simulink model "ROVSim_dp"  (R2020b)
settings: Solver=ode4  StartTime=0.0  StopTime=60  FixedStep=0.05  RelTol=1e-3
InitFcn:
  | initModelParam;
StopFcn:
  | %plotCoupled3DTrack;
libraries: pid_lib x9
settings Model: SimulationMode=accelerator  Creator=53549  LastModifiedBy=53549
settings DataIOCC: ReturnWorkspaceOutputs=off
settings DebuggingCC: ArithmeticOperatorsInVariantConditions=warning
settings SFSimCC: SimUseLocalCustomCode=off  CustomCodeUndefinedFunction=UseInterfaceOnly
settings RTWCC: RTWUseLocalCustomCode=off
settings CodeAppCC: StateflowObjectComments=on

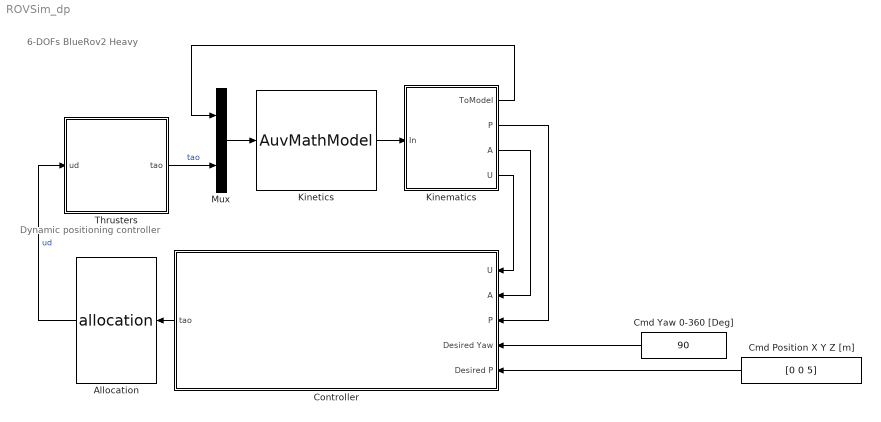
== system ROVSim_dp ==
  note: Dynamic positioning controller
  note: 6-DOFs BlueRov2 Heavy
  Allocation : MATLABFcn  MATLABFcn=allocation  OutputDimensions=8  OutputSignalType=real
  Cmd Position X Y Z [m] : Constant  Value=[0 0 5]
  Cmd Yaw 0-360 [Deg] : Constant  Value=90
  Controller : Subsystem
      mask Display: disp('Controller')
  Kinematics : Subsystem  mask{x0=10.00, y0=-0.00, z0=0.50, pitch0=0, yaw0=154.17, u0=0, flowDir=45, flowVel=0.2}
      mask prompts: x0 "Initiral x"; y0 "Initiral y"; z0 "Initiral z"; pitch0 "Initial pitch [Deg]"; yaw0 "Initial yaw [Deg]"; u0 "Initial velocity [m/s]"; flowDir "Flow direction [Deg]"; flowVel "Flow velocity [m/s]"
      mask DialogControl DescGroupVar Prompt: Kinematics
      mask DialogControl DescTextVar Prompt: Set kinematics information: AMV initial state, flow interference, etc
      mask DialogControl ParameterGroupVar Prompt: Initial state
      mask DialogControl Container3 Prompt: Flow
  Kinetics : MATLABFcn  MATLABFcn=AuvMathModel  OutputDimensions=6  OutputSignalType=real
      mask Display: image('blueRov.jpg')
  Mux : Mux  Inputs=2
  Thrusters : Subsystem  mask{dead_up=0.02, dead_low=-0.02, asym_gain=0.85}
      mask prompts: dead_up "Dead Zone Up Boundary [0, 1]"; dead_low "Dead Zone Low Boundary [-1, 0]"; asym_gain "Asymmetric Gain [0, 1]"
      mask DialogControl DescGroupVar Prompt: Thrusters model
      mask DialogControl DescTextVar Prompt: Thruster dead zone characteristic: When the input is near 0, the thruster does not rotate. Asymmetric characteristics of thrusters: With the same input, the thrust generated by reverse rotation of thrusters is less than that of forward rotation.
      mask Display: image('thruster.jfif');
  wires:
  Kinetics/1 -> Kinematics/1(In)
  Mux/1 -> Kinetics/1
  Kinematics/1(ToModel) -> Mux/1
  Kinematics/2(P) -> Controller/3(P)
  Thrusters/1(tao) -> Mux/2  "tao"
  Cmd Yaw 0-360 [Deg]/1 -> Controller/4(Desired Yaw)
  Cmd Position X Y Z [m]/1 -> Controller/5(Desired P)
  Controller/1(tao) -> Allocation/1
  Allocation/1 -> Thrusters/1(ud)  "ud"
  Kinematics/3(A) -> Controller/2(A)
  Kinematics/4(U) -> Controller/1(U)

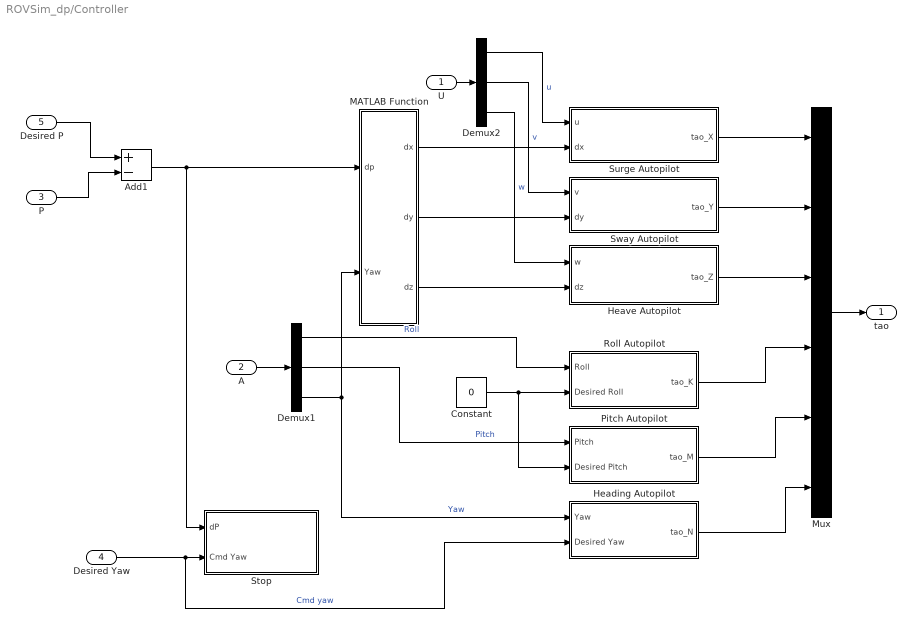
== system ROVSim_dp/Controller ==
  U : Inport
  A : Inport  Port=2
  P : Inport  Port=3
  Desired Yaw : Inport  Port=4
  Desired P : Inport  Port=5
  Add1 : Sum  Inputs=+-
  Constant : Constant  Value=0
  Demux1 : Demux  Outputs=3
  Demux2 : Demux  Outputs=3
  Heading Autopilot : Subsystem  mask{kp=0.2, ki=0, kd=0.2}
      mask DialogControl DescGroupVar Prompt: Heading Autopilot
      mask DialogControl DescTextVar Prompt: 设置PID增益。
      mask DialogControl ParameterGroupVar Prompt: PID Parameter
  Heave Autopilot : Subsystem
  MATLAB Function : MATLAB Function  TreatAsAtomicUnit=on
  Mux : Mux  Inputs=6
  Pitch Autopilot : Subsystem  mask{kp=5, ki=0, kd=0}
      mask DialogControl DescGroupVar Prompt: Heading Autopilot
      mask DialogControl DescTextVar Prompt: 设置PID增益。
      mask DialogControl ParameterGroupVar Prompt: PID Parameter
  Roll Autopilot : Subsystem  mask{kp=5, ki=0, kd=0}
      mask DialogControl DescGroupVar Prompt: Heading Autopilot
      mask DialogControl DescTextVar Prompt: 设置PID增益。
      mask DialogControl ParameterGroupVar Prompt: PID Parameter
  Stop : Subsystem
  Surge Autopilot : Subsystem
  Sway Autopilot : Subsystem
  tao : Outport
  wires:
  Demux1/3 -> Heading Autopilot/1(Yaw), MATLAB Function/2(Yaw)  "Yaw"
  Constant/1 -> Pitch Autopilot/2(Desired Pitch), Roll Autopilot/2(Desired Roll)
  Demux1/2 -> Pitch Autopilot/1(Pitch)  "Pitch"
  A/1 -> Demux1/1
  Desired P/1 -> Add1/1
  Add1/1 -> MATLAB Function/1(dp), Stop/1(dP)
  P/1 -> Add1/2
  Roll Autopilot/1(tao_K) -> Mux/4
  Pitch Autopilot/1(tao_M) -> Mux/5
  Heading Autopilot/1(tao_N) -> Mux/6
  Mux/1 -> tao/1
  Demux1/1 -> Roll Autopilot/1(Roll)  "Roll"
  U/1 -> Demux2/1
  Demux2/1 -> Surge Autopilot/1(u)  "u"
  MATLAB Function/1(dx) -> Surge Autopilot/2(dx)
  Surge Autopilot/1(tao_X) -> Mux/1
  Demux2/2 -> Sway Autopilot/1(v)  "v"
  MATLAB Function/2(dy) -> Sway Autopilot/2(dy)
  Sway Autopilot/1(tao_Y) -> Mux/2
  Demux2/3 -> Heave Autopilot/1(w)  "w"
  MATLAB Function/3(dz) -> Heave Autopilot/2(dz)
  Heave Autopilot/1(tao_Z) -> Mux/3
  Desired Yaw/1 -> Heading Autopilot/2(Desired Yaw), Stop/2(Cmd Yaw)  "Cmd yaw"

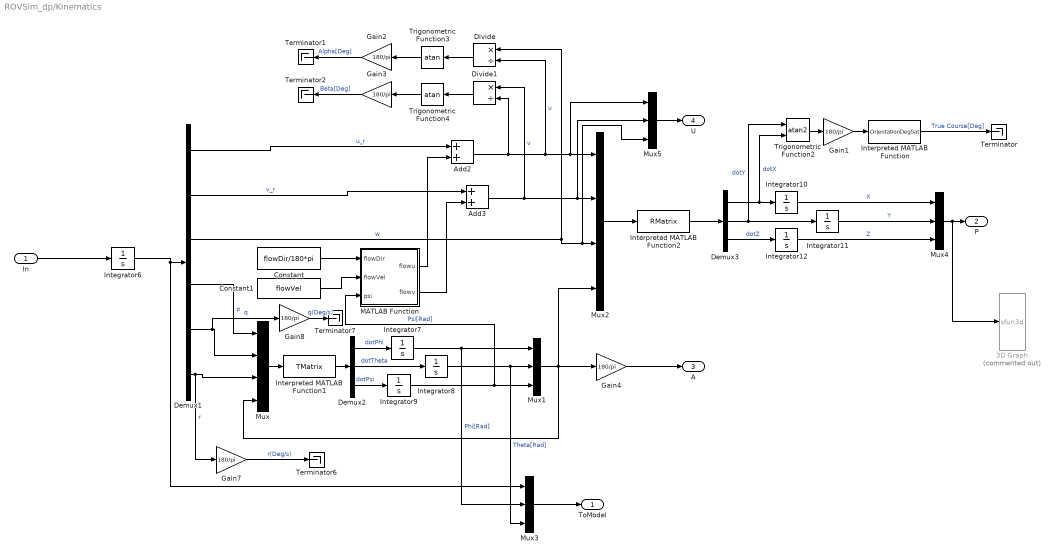
== system ROVSim_dp/Kinematics ==
  In : Inport
  3D Graph : S-Function  Commented=on  LoadFcn=if exist('sfun3d','file'), sfun3d([],[],[],'LoadBlock'); end  FunctionName=sfun3d  Parameters=ax,T,np,cp,gd,ls,mk,mx,hd,tb  SFunctionDeploymentMode=off  EnableBusSupport=off  mask(3D Graph){np=1, ax=[-15 15 -15 15 -5 20], mx=1e4, T=0.1, cp=[3 2 1], gd=on, hd=on, tb=off, ls=-, mk=none}
      mask prompts: np "Number of moving points (lines)"; ax "Range: [xmin xmax  ymin ymax zmin zmax]"; mx "Max number of points in each line"; T "Sampling Time"; cp "Camera position (use [0 0 1] for 2D XY view)"; gd "Grid (on|off)"; hd "HeadMarkers (on|off)"; tb "Toolbar (on|off)"; ls "LineStyle"; mk "LineMarker"
      mask help:
      | This block plots the position of several points in the XYZ space. The input contains the coordinates of all the points (x1,y1,z1,x2,y2,z2,...).
      | The number of moving points (lines), the XYZ ranges, sampling time, camera position, and grid (among other things) can be set as mask parameters.
      settings: CopyFcn=if exist('sfun3d','file'), sfun3d([],[],[],'CopyBlock'); end  DeleteFcn=if exist('sfun3d','file'), sfun3d([],[],[],'DeleteBlock'); end  NameChangeFcn=if exist('sfun3d','file'), sfun3d([],[],[],'NameChange'); end
      mask Help:
      | This block plots the position of several points in the XYZ space. The input contains the coordinates of all the points (x1,y1,z1,x2,y2,z2,...).
      | The number of moving points (lines), the XYZ ranges, sampling time, camera position, and grid (among other things) can be set as mask parameters.
      mask TypeOptions ls: - | -- | : | -. | none
      mask TypeOptions mk: none | . | + | o | * | x | square | diamond | v | ^ | > | < | pentagram | hexagram
      mask Display: plot([.05 .95 .95 .05 .05],[.45 .45 .95 .95 .45], 0.5+cos(0:0.1:2*pi)*0.3,0.7+sin(0:0.1:2*pi)*0.2)
  Add2 : Sum
  Add3 : Sum
  Constant : Constant  Value=flowDir/180*pi
  Constant1 : Constant  Value=flowVel
  Demux1 : Demux  Outputs=6
  Demux2 : Demux  Outputs=3
  Demux3 : Demux  Outputs=3
  Divide : Product  Inputs=*/
  Divide1 : Product  Inputs=*/
  Gain{1..4,7..8} (6 alike) : Gain  Gain=180/pi
  Integrator10 : Integrator  InitialCondition=x0
  Integrator11 : Integrator  InitialCondition=y0
  Integrator12 : Integrator  InitialCondition=z0
  Integrator6 : Integrator  InitialCondition=[u0; 0; 0; 0; 0; 0]
  Integrator7 : Integrator
  Integrator8 : Integrator
  Integrator9 : Integrator  InitialCondition=yaw0*pi/180  WrapState=on  WrappedStateUpperValue=6.2832  WrappedStateLowerValue=0
  Interpreted MATLAB Function : MATLABFcn  MATLABFcn=OrientationDegSat
  Interpreted MATLAB Function1 : MATLABFcn  MATLABFcn=TMatrix  OutputDimensions=3
  Interpreted MATLAB Function2 : MATLABFcn  MATLABFcn=RMatrix  OutputDimensions=3
  MATLAB Function : MATLAB Function  TreatAsAtomicUnit=on
  Mux : Mux
  Mux{1,3..5} (4 alike) : Mux  Inputs=3
  Mux2 : Mux
  Terminator{,1..2,6..7} (5 alike) : Terminator
  Trigonometric Function2 : Trigonometry  Operator=atan2
  Trigonometric Function3 : Trigonometry  Operator=atan
  Trigonometric Function4 : Trigonometry  Operator=atan
  ToModel : Outport
  P : Outport  Port=2
  A : Outport  Port=3
  U : Outport  Port=4
  wires:
  Constant/1 -> MATLAB Function/1(flowDir)
  Constant1/1 -> MATLAB Function/2(flowVel)
  Integrator6/1 -> Mux3/1, Demux1/1
  Demux1/4 -> Mux/1  "p"
  Demux1/5 -> Gain8/1, Mux/2  "q"
  Demux1/6 -> Gain7/1, Mux/3  "r"
  Mux/1 -> Interpreted MATLAB Function1/1
  Interpreted MATLAB Function1/1 -> Demux2/1
  Demux2/1 -> Integrator7/1  "dotPhi"
  Demux2/2 -> Integrator8/1  "dotTheta"
  Demux2/3 -> Integrator9/1  "dotPsi"
  Integrator9/1 -> MATLAB Function/3(psi), Mux1/3  "Psi[Rad]"
  Integrator7/1 -> Mux1/1, Mux3/2  "Phi[Rad]"
  Integrator8/1 -> Mux3/3, Mux1/2  "Theta[Rad]"
  Mux1/1 -> Gain4/1, Mux/4, Mux2/4
  Demux1/1 -> Add2/1  "u_r"
  Demux1/2 -> Add3/1  "v_r"
  Demux1/3 -> Mux5/3, Mux2/3, Divide/1  "w"
  Mux2/1 -> Interpreted MATLAB Function2/1
  Interpreted MATLAB Function2/1 -> Demux3/1
  Demux3/1 -> Trigonometric Function2/2, Integrator10/1  "dotX"
  Demux3/2 -> Trigonometric Function2/1, Integrator11/1  "dotY"
  Demux3/3 -> Integrator12/1  "dotZ"
  Integrator10/1 -> Mux4/1  "X"
  Integrator11/1 -> Mux4/2  "Y"
  Integrator12/1 -> Mux4/3  "Z"
  Gain2/1 -> Terminator1/1  "Alpha[Deg]"
  Trigonometric Function3/1 -> Gain2/1
  Divide/1 -> Trigonometric Function3/1
  Divide1/1 -> Trigonometric Function4/1
  Trigonometric Function4/1 -> Gain3/1
  Gain3/1 -> Terminator2/1  "Beta[Deg]"
  Gain1/1 -> Interpreted MATLAB Function/1
  Interpreted MATLAB Function/1 -> Terminator/1  "True Course[Deg]"
  Trigonometric Function2/1 -> Gain1/1
  Add2/1 -> Divide1/2, Divide/2, Mux5/1, Mux2/1  "u"
  Add3/1 -> Mux5/2, Mux2/2, Divide1/1  "v"
  MATLAB Function/1(flowu) -> Add2/2
  MATLAB Function/2(flowv) -> Add3/2
  Mux3/1 -> ToModel/1
  Mux4/1 -> 3D Graph/1, P/1
  In/1 -> Integrator6/1
  Gain7/1 -> Terminator6/1  "r(Deg/s)"
  Gain8/1 -> Terminator7/1  "q(Deg/s)"
  Gain4/1 -> A/1
  Mux5/1 -> U/1

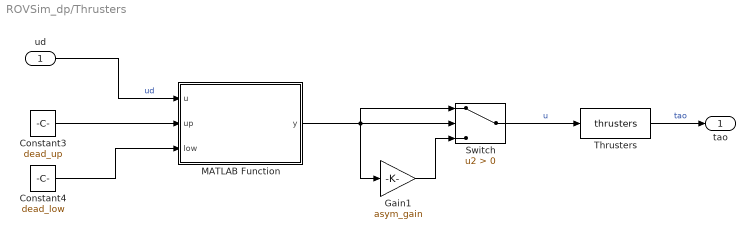
== system ROVSim_dp/Thrusters ==
  ud : Inport
  Constant3 : Constant  Value=dead_up
  Constant4 : Constant  Value=dead_low
  Gain1 : Gain  Gain=asym_gain
  MATLAB Function : MATLAB Function  TreatAsAtomicUnit=on
  Switch : Switch  Criteria=u2 > Threshold
  Thrusters : MATLABFcn  MATLABFcn=thrusters  OutputDimensions=6  OutputSignalType=real
  tao : Outport
  wires:
  Thrusters/1 -> tao/1  "tao"
  ud/1 -> MATLAB Function/1(u)  "ud"
  Gain1/1 -> Switch/3
  MATLAB Function/1(y) -> Switch/1, Gain1/1, Switch/2
  Constant4/1 -> MATLAB Function/3(low)
  Switch/1 -> Thrusters/1  "u"
  Constant3/1 -> MATLAB Function/2(up)

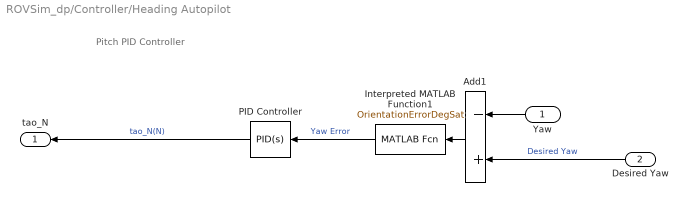
== system ROVSim_dp/Controller/Heading Autopilot ==
  note: Pitch PID Controller
  Yaw : Inport
  Desired Yaw : Inport  Port=2
  Add1 : Sum  Inputs=-+
  Interpreted MATLAB Function1 : MATLABFcn  MATLABFcn=OrientationErrorDegSat  OutputDimensions=1
  PID Controller : pid_lib/PID Controller  Controller=PID  Form=Parallel  TimeDomain=Continuous-time  UseExternalTs=off  SampleTime=-1  IntegratorMethod=Forward Euler  FilterMethod=Forward Euler  ControllerParametersSource=internal  P=kp  I=ki  D=kd  UseFilter=on  N=10  TunerSelectOption=Transfer Function Based (PID Tuner App)  InitialConditionSource=internal  InitialConditionForIntegrator=0  InitialConditionForFilter=0  DifferentiatorICPrevScaledInput=0  ExternalReset=none  TrackingMode=off  Kt=1  LimitOutput=on  SatLimitsSource=internal  UpperSaturationLimit=20  LowerSaturationLimit=-20  LinearizeAsGain=on  AntiWindupMode=none  Kb=1  POutMin=[]  POutMax=[]  IOutMin=[]  IOutMax=[]  DOutMin=[]  DOutMax=[]  NOutMin=[]  NOutMax=[]  SumOutMin=[]  SumOutMax=[]  SaturationOutMin=[]  SaturationOutMax=[]  PParamMin=[]  PParamMax=[]  IParamMin=[]  IParamMax=[]  DParamMin=[]  DParamMax=[]  NParamMin=[]  NParamMax=[]  KbParamMin=[]  KbParamMax=[]  KtParamMin=[]  KtParamMax=[]  KbOutMin=[]  KbOutMax=[]  KtOutMin=[]  KtOutMax=[]  IntegratorOutMin=[]  IntegratorOutMax=[]  FilterOutMin=[]  FilterOutMax=[]  SumI1OutMin=[]  SumI1OutMax=[]  SumI2OutMin=[]  SumI2OutMax=[]  SumI3OutMin=[]  SumI3OutMax=[]  SumI4OutMin=[]  SumI4OutMax=[]  SumDOutMin=[]  SumDOutMax=[]  DifferentiatorOutMin=[]  DifferentiatorOutMax=[]  FilterDiffOutCoefMin=[]  FilterDiffOutCoefMax=[]  ReciprocalOutMin=[]  ReciprocalOutMax=[]  SumDenOutMin=[]  SumDenOutMax=[]  SumNumOutMin=[]  SumNumOutMax=[]  DivideOutMin=[]  DivideOutMax=[]  UdiffTsProdOutMin=[]  UdiffTsProdOutMax=[]  NTsProdOutMin=[]  NTsProdOutMax=[]  UintegralTsProdOutMin=[]  UintegralTsProdOutMax=[]  UngainTsProdOutMin=[]  UngainTsProdOutMax=[]  IntegratorContinuousStateAttributes=''  IntegratorStateMustResolveToSignalObject=off  IntegratorRTWStateStorageClass=Auto  FilterContinuousStateAttributes=''  FilterStateMustResolveToSignalObject=off  FilterRTWStateStorageClass=Auto  ParallelPVariant=InternalParameters  IdealPVariant=Disabled  IVariant=InternalParameters  DVariant=InternalParameters  IntegratorVariant=Continuous  SatVariant=Enabled  AWVariant=Passthrough  PCopyVariant=Disabled  TRVariant=Disabled  FdbkBlocksVariant=Forward  IdealPFdbkVariant=Disabled  SatFdbkVariant=Disabled  DerivativeFilterVariant=ContFilter  NVariant=InternalParameters  NCopyVariant=Disabled  FilterICVariant=InternalICsFilter  IntegratorICVariant=InternalICs  ExternalResetVariant=Disabled  TRSumVariant=Passthrough  SumFdbkVariant=Disabled  SumVariant=Sum_PID  TsampFilterVariant=InternalTs  TsampNgainVariant=Passthrough  TsampIntegralVariant=Passthrough  ExternalSaturationOutDataTypeStr=Inherit: Same as second input
  tao_N : Outport
  wires:
  Yaw/1 -> Add1/1
  PID Controller/1 -> tao_N/1  "tao_N(N)"
  Add1/1 -> Interpreted MATLAB Function1/1
  Desired Yaw/1 -> Add1/2  "Desired Yaw"
  Interpreted MATLAB Function1/1 -> PID Controller/1  "Yaw Error"

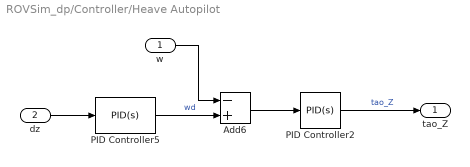
== system ROVSim_dp/Controller/Heave Autopilot ==
  w : Inport
  dz : Inport  Port=2
  Add6 : Sum  Inputs=-+
  PID Controller2 : pid_lib/PID Controller  Controller=PID  Form=Parallel  TimeDomain=Continuous-time  UseExternalTs=off  SampleTime=-1  IntegratorMethod=Forward Euler  FilterMethod=Forward Euler  ControllerParametersSource=internal  P=40  I=0.5  D=0  UseFilter=on  N=100  TunerSelectOption=Transfer Function Based (PID Tuner App)  InitialConditionSource=internal  InitialConditionForIntegrator=0  InitialConditionForFilter=0  DifferentiatorICPrevScaledInput=0  ExternalReset=none  TrackingMode=off  Kt=1  LimitOutput=off  SatLimitsSource=internal  UpperSaturationLimit=inf  LowerSaturationLimit=-inf  LinearizeAsGain=on  AntiWindupMode=none  Kb=1  POutMin=[]  POutMax=[]  IOutMin=[]  IOutMax=[]  DOutMin=[]  DOutMax=[]  NOutMin=[]  NOutMax=[]  SumOutMin=[]  SumOutMax=[]  SaturationOutMin=[]  SaturationOutMax=[]  PParamMin=[]  PParamMax=[]  IParamMin=[]  IParamMax=[]  DParamMin=[]  DParamMax=[]  NParamMin=[]  NParamMax=[]  KbParamMin=[]  KbParamMax=[]  KtParamMin=[]  KtParamMax=[]  KbOutMin=[]  KbOutMax=[]  KtOutMin=[]  KtOutMax=[]  IntegratorOutMin=[]  IntegratorOutMax=[]  FilterOutMin=[]  FilterOutMax=[]  SumI1OutMin=[]  SumI1OutMax=[]  SumI2OutMin=[]  SumI2OutMax=[]  SumI3OutMin=[]  SumI3OutMax=[]  SumI4OutMin=[]  SumI4OutMax=[]  SumDOutMin=[]  SumDOutMax=[]  DifferentiatorOutMin=[]  DifferentiatorOutMax=[]  FilterDiffOutCoefMin=[]  FilterDiffOutCoefMax=[]  ReciprocalOutMin=[]  ReciprocalOutMax=[]  SumDenOutMin=[]  SumDenOutMax=[]  SumNumOutMin=[]  SumNumOutMax=[]  DivideOutMin=[]  DivideOutMax=[]  UdiffTsProdOutMin=[]  UdiffTsProdOutMax=[]  NTsProdOutMin=[]  NTsProdOutMax=[]  UintegralTsProdOutMin=[]  UintegralTsProdOutMax=[]  UngainTsProdOutMin=[]  UngainTsProdOutMax=[]  IntegratorContinuousStateAttributes=''  IntegratorStateMustResolveToSignalObject=off  IntegratorRTWStateStorageClass=Auto  FilterContinuousStateAttributes=''  FilterStateMustResolveToSignalObject=off  FilterRTWStateStorageClass=Auto  ParallelPVariant=InternalParameters  IdealPVariant=Disabled  IVariant=InternalParameters  DVariant=InternalParameters  IntegratorVariant=Continuous  SatVariant=Disabled  AWVariant=Passthrough  PCopyVariant=Disabled  TRVariant=Disabled  FdbkBlocksVariant=Forward  IdealPFdbkVariant=Disabled  SatFdbkVariant=Disabled  DerivativeFilterVariant=ContFilter  NVariant=InternalParameters  NCopyVariant=Disabled  FilterICVariant=InternalICsFilter  IntegratorICVariant=InternalICs  ExternalResetVariant=Disabled  TRSumVariant=Passthrough  SumFdbkVariant=Disabled  SumVariant=Sum_PID  TsampFilterVariant=InternalTs  TsampNgainVariant=Passthrough  TsampIntegralVariant=Passthrough  ExternalSaturationOutDataTypeStr=Inherit: Same as second input
  PID Controller5 : pid_lib/PID Controller  Controller=PID  Form=Parallel  TimeDomain=Continuous-time  UseExternalTs=off  SampleTime=-1  IntegratorMethod=Forward Euler  FilterMethod=Forward Euler  ControllerParametersSource=internal  P=0.5  I=0  D=0  UseFilter=on  N=100  TunerSelectOption=Transfer Function Based (PID Tuner App)  InitialConditionSource=internal  InitialConditionForIntegrator=0  InitialConditionForFilter=0  DifferentiatorICPrevScaledInput=0  ExternalReset=none  TrackingMode=off  Kt=1  LimitOutput=on  SatLimitsSource=internal  UpperSaturationLimit=1  LowerSaturationLimit=-1  LinearizeAsGain=on  AntiWindupMode=none  Kb=1  POutMin=[]  POutMax=[]  IOutMin=[]  IOutMax=[]  DOutMin=[]  DOutMax=[]  NOutMin=[]  NOutMax=[]  SumOutMin=[]  SumOutMax=[]  SaturationOutMin=[]  SaturationOutMax=[]  PParamMin=[]  PParamMax=[]  IParamMin=[]  IParamMax=[]  DParamMin=[]  DParamMax=[]  NParamMin=[]  NParamMax=[]  KbParamMin=[]  KbParamMax=[]  KtParamMin=[]  KtParamMax=[]  KbOutMin=[]  KbOutMax=[]  KtOutMin=[]  KtOutMax=[]  IntegratorOutMin=[]  IntegratorOutMax=[]  FilterOutMin=[]  FilterOutMax=[]  SumI1OutMin=[]  SumI1OutMax=[]  SumI2OutMin=[]  SumI2OutMax=[]  SumI3OutMin=[]  SumI3OutMax=[]  SumI4OutMin=[]  SumI4OutMax=[]  SumDOutMin=[]  SumDOutMax=[]  DifferentiatorOutMin=[]  DifferentiatorOutMax=[]  FilterDiffOutCoefMin=[]  FilterDiffOutCoefMax=[]  ReciprocalOutMin=[]  ReciprocalOutMax=[]  SumDenOutMin=[]  SumDenOutMax=[]  SumNumOutMin=[]  SumNumOutMax=[]  DivideOutMin=[]  DivideOutMax=[]  UdiffTsProdOutMin=[]  UdiffTsProdOutMax=[]  NTsProdOutMin=[]  NTsProdOutMax=[]  UintegralTsProdOutMin=[]  UintegralTsProdOutMax=[]  UngainTsProdOutMin=[]  UngainTsProdOutMax=[]  IntegratorContinuousStateAttributes=''  IntegratorStateMustResolveToSignalObject=off  IntegratorRTWStateStorageClass=Auto  FilterContinuousStateAttributes=''  FilterStateMustResolveToSignalObject=off  FilterRTWStateStorageClass=Auto  ParallelPVariant=InternalParameters  IdealPVariant=Disabled  IVariant=InternalParameters  DVariant=InternalParameters  IntegratorVariant=Continuous  SatVariant=Enabled  AWVariant=Passthrough  PCopyVariant=Disabled  TRVariant=Disabled  FdbkBlocksVariant=Forward  IdealPFdbkVariant=Disabled  SatFdbkVariant=Disabled  DerivativeFilterVariant=ContFilter  NVariant=InternalParameters  NCopyVariant=Disabled  FilterICVariant=InternalICsFilter  IntegratorICVariant=InternalICs  ExternalResetVariant=Disabled  TRSumVariant=Passthrough  SumFdbkVariant=Disabled  SumVariant=Sum_PID  TsampFilterVariant=InternalTs  TsampNgainVariant=Passthrough  TsampIntegralVariant=Passthrough  ExternalSaturationOutDataTypeStr=Inherit: Same as second input
  tao_Z : Outport
  wires:
  Add6/1 -> PID Controller2/1
  PID Controller5/1 -> Add6/2  "wd"
  dz/1 -> PID Controller5/1
  PID Controller2/1 -> tao_Z/1  "tao_Z"
  w/1 -> Add6/1

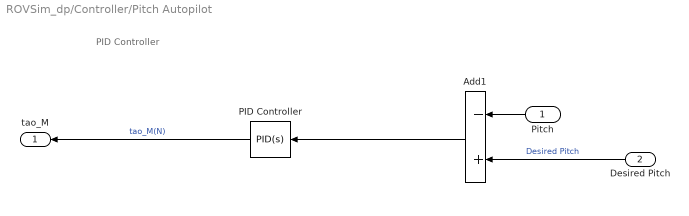
== system ROVSim_dp/Controller/Pitch Autopilot ==
  note: PID Controller
  Pitch : Inport
  Desired Pitch : Inport  Port=2
  Add1 : Sum  Inputs=-+
  PID Controller : pid_lib/PID Controller  Controller=PID  Form=Parallel  TimeDomain=Continuous-time  UseExternalTs=off  SampleTime=-1  IntegratorMethod=Forward Euler  FilterMethod=Forward Euler  ControllerParametersSource=internal  P=kp  I=ki  D=kd  UseFilter=on  N=10  TunerSelectOption=Transfer Function Based (PID Tuner App)  InitialConditionSource=internal  InitialConditionForIntegrator=0  InitialConditionForFilter=0  DifferentiatorICPrevScaledInput=0  ExternalReset=none  TrackingMode=off  Kt=1  LimitOutput=on  SatLimitsSource=internal  UpperSaturationLimit=20  LowerSaturationLimit=-20  LinearizeAsGain=on  AntiWindupMode=none  Kb=1  POutMin=[]  POutMax=[]  IOutMin=[]  IOutMax=[]  DOutMin=[]  DOutMax=[]  NOutMin=[]  NOutMax=[]  SumOutMin=[]  SumOutMax=[]  SaturationOutMin=[]  SaturationOutMax=[]  PParamMin=[]  PParamMax=[]  IParamMin=[]  IParamMax=[]  DParamMin=[]  DParamMax=[]  NParamMin=[]  NParamMax=[]  KbParamMin=[]  KbParamMax=[]  KtParamMin=[]  KtParamMax=[]  KbOutMin=[]  KbOutMax=[]  KtOutMin=[]  KtOutMax=[]  IntegratorOutMin=[]  IntegratorOutMax=[]  FilterOutMin=[]  FilterOutMax=[]  SumI1OutMin=[]  SumI1OutMax=[]  SumI2OutMin=[]  SumI2OutMax=[]  SumI3OutMin=[]  SumI3OutMax=[]  SumI4OutMin=[]  SumI4OutMax=[]  SumDOutMin=[]  SumDOutMax=[]  DifferentiatorOutMin=[]  DifferentiatorOutMax=[]  FilterDiffOutCoefMin=[]  FilterDiffOutCoefMax=[]  ReciprocalOutMin=[]  ReciprocalOutMax=[]  SumDenOutMin=[]  SumDenOutMax=[]  SumNumOutMin=[]  SumNumOutMax=[]  DivideOutMin=[]  DivideOutMax=[]  UdiffTsProdOutMin=[]  UdiffTsProdOutMax=[]  NTsProdOutMin=[]  NTsProdOutMax=[]  UintegralTsProdOutMin=[]  UintegralTsProdOutMax=[]  UngainTsProdOutMin=[]  UngainTsProdOutMax=[]  IntegratorContinuousStateAttributes=''  IntegratorStateMustResolveToSignalObject=off  IntegratorRTWStateStorageClass=Auto  FilterContinuousStateAttributes=''  FilterStateMustResolveToSignalObject=off  FilterRTWStateStorageClass=Auto  ParallelPVariant=InternalParameters  IdealPVariant=Disabled  IVariant=InternalParameters  DVariant=InternalParameters  IntegratorVariant=Continuous  SatVariant=Enabled  AWVariant=Passthrough  PCopyVariant=Disabled  TRVariant=Disabled  FdbkBlocksVariant=Forward  IdealPFdbkVariant=Disabled  SatFdbkVariant=Disabled  DerivativeFilterVariant=ContFilter  NVariant=InternalParameters  NCopyVariant=Disabled  FilterICVariant=InternalICsFilter  IntegratorICVariant=InternalICs  ExternalResetVariant=Disabled  TRSumVariant=Passthrough  SumFdbkVariant=Disabled  SumVariant=Sum_PID  TsampFilterVariant=InternalTs  TsampNgainVariant=Passthrough  TsampIntegralVariant=Passthrough  ExternalSaturationOutDataTypeStr=Inherit: Same as second input
  tao_M : Outport
  wires:
  Add1/1 -> PID Controller/1
  Desired Pitch/1 -> Add1/2  "Desired Pitch"
  PID Controller/1 -> tao_M/1  "tao_M(N)"
  Pitch/1 -> Add1/1

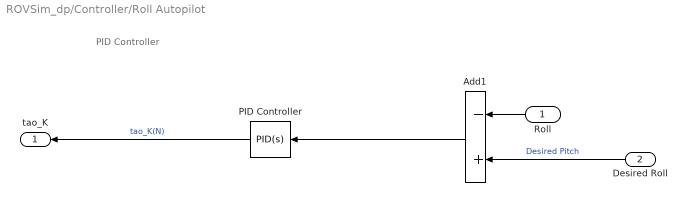
== system ROVSim_dp/Controller/Roll Autopilot ==
  note: PID Controller
  Roll : Inport
  Desired Roll : Inport  Port=2
  Add1 : Sum  Inputs=-+
  PID Controller : pid_lib/PID Controller  Controller=PID  Form=Parallel  TimeDomain=Continuous-time  UseExternalTs=off  SampleTime=-1  IntegratorMethod=Forward Euler  FilterMethod=Forward Euler  ControllerParametersSource=internal  P=kp  I=ki  D=kd  UseFilter=on  N=10  TunerSelectOption=Transfer Function Based (PID Tuner App)  InitialConditionSource=internal  InitialConditionForIntegrator=0  InitialConditionForFilter=0  DifferentiatorICPrevScaledInput=0  ExternalReset=none  TrackingMode=off  Kt=1  LimitOutput=on  SatLimitsSource=internal  UpperSaturationLimit=20  LowerSaturationLimit=-20  LinearizeAsGain=on  AntiWindupMode=none  Kb=1  POutMin=[]  POutMax=[]  IOutMin=[]  IOutMax=[]  DOutMin=[]  DOutMax=[]  NOutMin=[]  NOutMax=[]  SumOutMin=[]  SumOutMax=[]  SaturationOutMin=[]  SaturationOutMax=[]  PParamMin=[]  PParamMax=[]  IParamMin=[]  IParamMax=[]  DParamMin=[]  DParamMax=[]  NParamMin=[]  NParamMax=[]  KbParamMin=[]  KbParamMax=[]  KtParamMin=[]  KtParamMax=[]  KbOutMin=[]  KbOutMax=[]  KtOutMin=[]  KtOutMax=[]  IntegratorOutMin=[]  IntegratorOutMax=[]  FilterOutMin=[]  FilterOutMax=[]  SumI1OutMin=[]  SumI1OutMax=[]  SumI2OutMin=[]  SumI2OutMax=[]  SumI3OutMin=[]  SumI3OutMax=[]  SumI4OutMin=[]  SumI4OutMax=[]  SumDOutMin=[]  SumDOutMax=[]  DifferentiatorOutMin=[]  DifferentiatorOutMax=[]  FilterDiffOutCoefMin=[]  FilterDiffOutCoefMax=[]  ReciprocalOutMin=[]  ReciprocalOutMax=[]  SumDenOutMin=[]  SumDenOutMax=[]  SumNumOutMin=[]  SumNumOutMax=[]  DivideOutMin=[]  DivideOutMax=[]  UdiffTsProdOutMin=[]  UdiffTsProdOutMax=[]  NTsProdOutMin=[]  NTsProdOutMax=[]  UintegralTsProdOutMin=[]  UintegralTsProdOutMax=[]  UngainTsProdOutMin=[]  UngainTsProdOutMax=[]  IntegratorContinuousStateAttributes=''  IntegratorStateMustResolveToSignalObject=off  IntegratorRTWStateStorageClass=Auto  FilterContinuousStateAttributes=''  FilterStateMustResolveToSignalObject=off  FilterRTWStateStorageClass=Auto  ParallelPVariant=InternalParameters  IdealPVariant=Disabled  IVariant=InternalParameters  DVariant=InternalParameters  IntegratorVariant=Continuous  SatVariant=Enabled  AWVariant=Passthrough  PCopyVariant=Disabled  TRVariant=Disabled  FdbkBlocksVariant=Forward  IdealPFdbkVariant=Disabled  SatFdbkVariant=Disabled  DerivativeFilterVariant=ContFilter  NVariant=InternalParameters  NCopyVariant=Disabled  FilterICVariant=InternalICsFilter  IntegratorICVariant=InternalICs  ExternalResetVariant=Disabled  TRSumVariant=Passthrough  SumFdbkVariant=Disabled  SumVariant=Sum_PID  TsampFilterVariant=InternalTs  TsampNgainVariant=Passthrough  TsampIntegralVariant=Passthrough  ExternalSaturationOutDataTypeStr=Inherit: Same as second input
  tao_K : Outport
  wires:
  Roll/1 -> Add1/1
  PID Controller/1 -> tao_K/1  "tao_K(N)"
  Desired Roll/1 -> Add1/2  "Desired Pitch"
  Add1/1 -> PID Controller/1

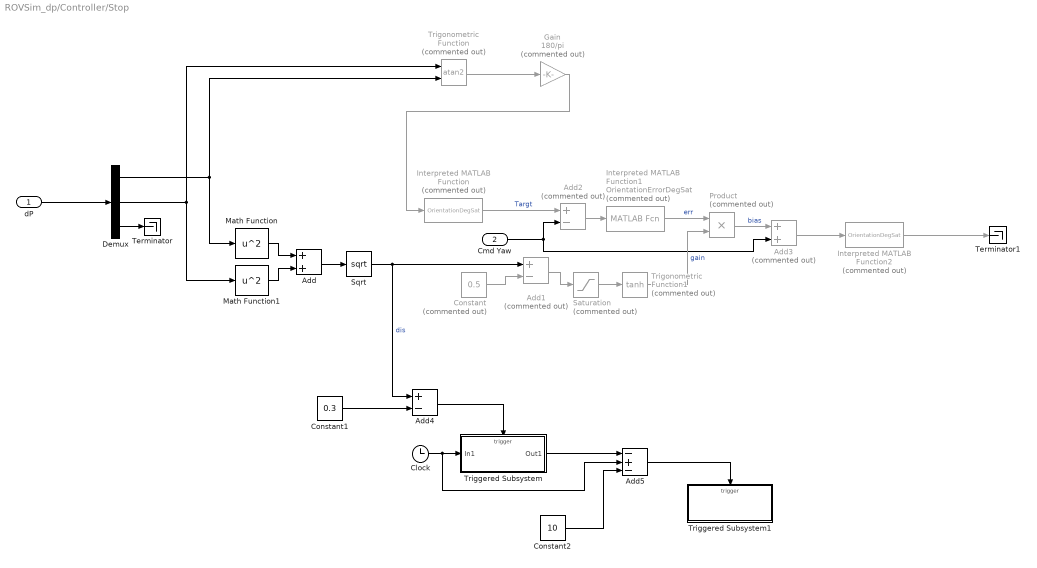
== system ROVSim_dp/Controller/Stop ==
  dP : Inport
  Cmd Yaw : Inport  Port=2
  Add : Sum
  Add1 : Sum  Commented=on  Inputs=+-
  Add2 : Sum  Commented=on  Inputs=+-
  Add3 : Sum  Commented=on
  Add4 : Sum  Inputs=+-
  Add5 : Sum  Inputs=-+-
  Clock : Clock
  Constant : Constant  Commented=on  Value=0.5
  Constant1 : Constant  Value=0.3
  Constant2 : Constant  Value=10
  Demux : Demux  Outputs=3
  Gain : Gain  Commented=on  Gain=180/pi
  Interpreted MATLAB Function : MATLABFcn  Commented=on  MATLABFcn=OrientationDegSat  OutputDimensions=1
  Interpreted MATLAB Function1 : MATLABFcn  Commented=on  MATLABFcn=OrientationErrorDegSat  OutputDimensions=1
  Interpreted MATLAB Function2 : MATLABFcn  Commented=on  MATLABFcn=OrientationDegSat  OutputDimensions=1
  Math Function : Math  Operator=square  SaturateOnIntegerOverflow=on
  Math Function1 : Math  Operator=square  SaturateOnIntegerOverflow=on
  Product : Product  Commented=on
  Saturation : Saturate  Commented=on  UpperLimit=inf  LowerLimit=0
  Sqrt : Sqrt  SaturateOnIntegerOverflow=on
  Terminator : Terminator
  Terminator1 : Terminator
  Triggered Subsystem : Subsystem  TreatAsAtomicUnit=on
  Triggered Subsystem1 : Subsystem  TreatAsAtomicUnit=on
  Trigonometric Function : Trigonometry  Commented=on  Operator=atan2
  Trigonometric Function1 : Trigonometry  Commented=on  Operator=tanh
  wires:
  Math Function/1 -> Add/1
  Product/1 -> Add3/1  "bias"
  Interpreted MATLAB Function/1 -> Add2/1  "Targt"
  Cmd Yaw/1 -> Add2/2, Add3/2
  dP/1 -> Demux/1
  Gain/1 -> Interpreted MATLAB Function/1
  Demux/1 -> Math Function/1, Trigonometric Function/2
  Add3/1 -> Interpreted MATLAB Function2/1
  Interpreted MATLAB Function1/1 -> Product/1  "err"
  Demux/3 -> Terminator/1
  Trigonometric Function/1 -> Gain/1
  Demux/2 -> Math Function1/1, Trigonometric Function/1
  Add/1 -> Sqrt/1
  Sqrt/1 -> Add4/1, Add1/1  "dis"
  Add2/1 -> Interpreted MATLAB Function1/1
  Trigonometric Function1/1 -> Product/2  "gain"
  Math Function1/1 -> Add/2
  Interpreted MATLAB Function2/1 -> Terminator1/1
  Constant/1 -> Add1/2
  Add1/1 -> Saturation/1
  Saturation/1 -> Trigonometric Function1/1
  Constant1/1 -> Add4/2
  Add4/1 -> Triggered Subsystem/Trigger
  Clock/1 -> Add5/2, Triggered Subsystem/1(In1)
  Triggered Subsystem/1(Out1) -> Add5/1
  Add5/1 -> Triggered Subsystem1/Trigger
  Constant2/1 -> Add5/3

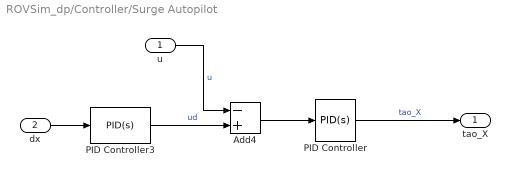
== system ROVSim_dp/Controller/Surge Autopilot ==
  u : Inport
  dx : Inport  Port=2
  Add4 : Sum  Inputs=-+
  PID Controller : pid_lib/PID Controller  Controller=PID  Form=Parallel  TimeDomain=Continuous-time  UseExternalTs=off  SampleTime=-1  IntegratorMethod=Forward Euler  FilterMethod=Forward Euler  ControllerParametersSource=internal  P=20  I=0  D=0  UseFilter=on  N=100  TunerSelectOption=Transfer Function Based (PID Tuner App)  InitialConditionSource=internal  InitialConditionForIntegrator=0  InitialConditionForFilter=0  DifferentiatorICPrevScaledInput=0  ExternalReset=none  TrackingMode=off  Kt=1  LimitOutput=off  SatLimitsSource=internal  UpperSaturationLimit=inf  LowerSaturationLimit=-inf  LinearizeAsGain=on  AntiWindupMode=none  Kb=1  POutMin=[]  POutMax=[]  IOutMin=[]  IOutMax=[]  DOutMin=[]  DOutMax=[]  NOutMin=[]  NOutMax=[]  SumOutMin=[]  SumOutMax=[]  SaturationOutMin=[]  SaturationOutMax=[]  PParamMin=[]  PParamMax=[]  IParamMin=[]  IParamMax=[]  DParamMin=[]  DParamMax=[]  NParamMin=[]  NParamMax=[]  KbParamMin=[]  KbParamMax=[]  KtParamMin=[]  KtParamMax=[]  KbOutMin=[]  KbOutMax=[]  KtOutMin=[]  KtOutMax=[]  IntegratorOutMin=[]  IntegratorOutMax=[]  FilterOutMin=[]  FilterOutMax=[]  SumI1OutMin=[]  SumI1OutMax=[]  SumI2OutMin=[]  SumI2OutMax=[]  SumI3OutMin=[]  SumI3OutMax=[]  SumI4OutMin=[]  SumI4OutMax=[]  SumDOutMin=[]  SumDOutMax=[]  DifferentiatorOutMin=[]  DifferentiatorOutMax=[]  FilterDiffOutCoefMin=[]  FilterDiffOutCoefMax=[]  ReciprocalOutMin=[]  ReciprocalOutMax=[]  SumDenOutMin=[]  SumDenOutMax=[]  SumNumOutMin=[]  SumNumOutMax=[]  DivideOutMin=[]  DivideOutMax=[]  UdiffTsProdOutMin=[]  UdiffTsProdOutMax=[]  NTsProdOutMin=[]  NTsProdOutMax=[]  UintegralTsProdOutMin=[]  UintegralTsProdOutMax=[]  UngainTsProdOutMin=[]  UngainTsProdOutMax=[]  IntegratorContinuousStateAttributes=''  IntegratorStateMustResolveToSignalObject=off  IntegratorRTWStateStorageClass=Auto  FilterContinuousStateAttributes=''  FilterStateMustResolveToSignalObject=off  FilterRTWStateStorageClass=Auto  ParallelPVariant=InternalParameters  IdealPVariant=Disabled  IVariant=InternalParameters  DVariant=InternalParameters  IntegratorVariant=Continuous  SatVariant=Disabled  AWVariant=Passthrough  PCopyVariant=Disabled  TRVariant=Disabled  FdbkBlocksVariant=Forward  IdealPFdbkVariant=Disabled  SatFdbkVariant=Disabled  DerivativeFilterVariant=ContFilter  NVariant=InternalParameters  NCopyVariant=Disabled  FilterICVariant=InternalICsFilter  IntegratorICVariant=InternalICs  ExternalResetVariant=Disabled  TRSumVariant=Passthrough  SumFdbkVariant=Disabled  SumVariant=Sum_PID  TsampFilterVariant=InternalTs  TsampNgainVariant=Passthrough  TsampIntegralVariant=Passthrough  ExternalSaturationOutDataTypeStr=Inherit: Same as second input
  PID Controller3 : pid_lib/PID Controller  Controller=PID  Form=Parallel  TimeDomain=Continuous-time  UseExternalTs=off  SampleTime=-1  IntegratorMethod=Forward Euler  FilterMethod=Forward Euler  ControllerParametersSource=internal  P=0.5  I=0  D=0  UseFilter=on  N=100  TunerSelectOption=Transfer Function Based (PID Tuner App)  InitialConditionSource=internal  InitialConditionForIntegrator=0  InitialConditionForFilter=0  DifferentiatorICPrevScaledInput=0  ExternalReset=none  TrackingMode=off  Kt=1  LimitOutput=on  SatLimitsSource=internal  UpperSaturationLimit=1  LowerSaturationLimit=-1  LinearizeAsGain=on  AntiWindupMode=none  Kb=1  POutMin=[]  POutMax=[]  IOutMin=[]  IOutMax=[]  DOutMin=[]  DOutMax=[]  NOutMin=[]  NOutMax=[]  SumOutMin=[]  SumOutMax=[]  SaturationOutMin=[]  SaturationOutMax=[]  PParamMin=[]  PParamMax=[]  IParamMin=[]  IParamMax=[]  DParamMin=[]  DParamMax=[]  NParamMin=[]  NParamMax=[]  KbParamMin=[]  KbParamMax=[]  KtParamMin=[]  KtParamMax=[]  KbOutMin=[]  KbOutMax=[]  KtOutMin=[]  KtOutMax=[]  IntegratorOutMin=[]  IntegratorOutMax=[]  FilterOutMin=[]  FilterOutMax=[]  SumI1OutMin=[]  SumI1OutMax=[]  SumI2OutMin=[]  SumI2OutMax=[]  SumI3OutMin=[]  SumI3OutMax=[]  SumI4OutMin=[]  SumI4OutMax=[]  SumDOutMin=[]  SumDOutMax=[]  DifferentiatorOutMin=[]  DifferentiatorOutMax=[]  FilterDiffOutCoefMin=[]  FilterDiffOutCoefMax=[]  ReciprocalOutMin=[]  ReciprocalOutMax=[]  SumDenOutMin=[]  SumDenOutMax=[]  SumNumOutMin=[]  SumNumOutMax=[]  DivideOutMin=[]  DivideOutMax=[]  UdiffTsProdOutMin=[]  UdiffTsProdOutMax=[]  NTsProdOutMin=[]  NTsProdOutMax=[]  UintegralTsProdOutMin=[]  UintegralTsProdOutMax=[]  UngainTsProdOutMin=[]  UngainTsProdOutMax=[]  IntegratorContinuousStateAttributes=''  IntegratorStateMustResolveToSignalObject=off  IntegratorRTWStateStorageClass=Auto  FilterContinuousStateAttributes=''  FilterStateMustResolveToSignalObject=off  FilterRTWStateStorageClass=Auto  ParallelPVariant=InternalParameters  IdealPVariant=Disabled  IVariant=InternalParameters  DVariant=InternalParameters  IntegratorVariant=Continuous  SatVariant=Enabled  AWVariant=Passthrough  PCopyVariant=Disabled  TRVariant=Disabled  FdbkBlocksVariant=Forward  IdealPFdbkVariant=Disabled  SatFdbkVariant=Disabled  DerivativeFilterVariant=ContFilter  NVariant=InternalParameters  NCopyVariant=Disabled  FilterICVariant=InternalICsFilter  IntegratorICVariant=InternalICs  ExternalResetVariant=Disabled  TRSumVariant=Passthrough  SumFdbkVariant=Disabled  SumVariant=Sum_PID  TsampFilterVariant=InternalTs  TsampNgainVariant=Passthrough  TsampIntegralVariant=Passthrough  ExternalSaturationOutDataTypeStr=Inherit: Same as second input
  tao_X : Outport
  wires:
  PID Controller/1 -> tao_X/1  "tao_X"
  Add4/1 -> PID Controller/1
  PID Controller3/1 -> Add4/2  "ud"
  dx/1 -> PID Controller3/1
  u/1 -> Add4/1  "u"

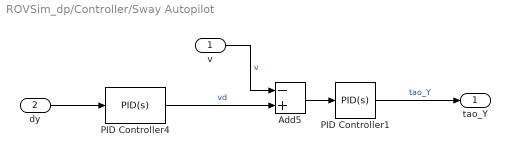
== system ROVSim_dp/Controller/Sway Autopilot ==
  v : Inport
  dy : Inport  Port=2
  Add5 : Sum  Inputs=-+
  PID Controller1 : pid_lib/PID Controller  Controller=PID  Form=Parallel  TimeDomain=Continuous-time  UseExternalTs=off  SampleTime=-1  IntegratorMethod=Forward Euler  FilterMethod=Forward Euler  ControllerParametersSource=internal  P=20  I=0  D=0  UseFilter=on  N=100  TunerSelectOption=Transfer Function Based (PID Tuner App)  InitialConditionSource=internal  InitialConditionForIntegrator=0  InitialConditionForFilter=0  DifferentiatorICPrevScaledInput=0  ExternalReset=none  TrackingMode=off  Kt=1  LimitOutput=off  SatLimitsSource=internal  UpperSaturationLimit=inf  LowerSaturationLimit=-inf  LinearizeAsGain=on  AntiWindupMode=none  Kb=1  POutMin=[]  POutMax=[]  IOutMin=[]  IOutMax=[]  DOutMin=[]  DOutMax=[]  NOutMin=[]  NOutMax=[]  SumOutMin=[]  SumOutMax=[]  SaturationOutMin=[]  SaturationOutMax=[]  PParamMin=[]  PParamMax=[]  IParamMin=[]  IParamMax=[]  DParamMin=[]  DParamMax=[]  NParamMin=[]  NParamMax=[]  KbParamMin=[]  KbParamMax=[]  KtParamMin=[]  KtParamMax=[]  KbOutMin=[]  KbOutMax=[]  KtOutMin=[]  KtOutMax=[]  IntegratorOutMin=[]  IntegratorOutMax=[]  FilterOutMin=[]  FilterOutMax=[]  SumI1OutMin=[]  SumI1OutMax=[]  SumI2OutMin=[]  SumI2OutMax=[]  SumI3OutMin=[]  SumI3OutMax=[]  SumI4OutMin=[]  SumI4OutMax=[]  SumDOutMin=[]  SumDOutMax=[]  DifferentiatorOutMin=[]  DifferentiatorOutMax=[]  FilterDiffOutCoefMin=[]  FilterDiffOutCoefMax=[]  ReciprocalOutMin=[]  ReciprocalOutMax=[]  SumDenOutMin=[]  SumDenOutMax=[]  SumNumOutMin=[]  SumNumOutMax=[]  DivideOutMin=[]  DivideOutMax=[]  UdiffTsProdOutMin=[]  UdiffTsProdOutMax=[]  NTsProdOutMin=[]  NTsProdOutMax=[]  UintegralTsProdOutMin=[]  UintegralTsProdOutMax=[]  UngainTsProdOutMin=[]  UngainTsProdOutMax=[]  IntegratorContinuousStateAttributes=''  IntegratorStateMustResolveToSignalObject=off  IntegratorRTWStateStorageClass=Auto  FilterContinuousStateAttributes=''  FilterStateMustResolveToSignalObject=off  FilterRTWStateStorageClass=Auto  ParallelPVariant=InternalParameters  IdealPVariant=Disabled  IVariant=InternalParameters  DVariant=InternalParameters  IntegratorVariant=Continuous  SatVariant=Disabled  AWVariant=Passthrough  PCopyVariant=Disabled  TRVariant=Disabled  FdbkBlocksVariant=Forward  IdealPFdbkVariant=Disabled  SatFdbkVariant=Disabled  DerivativeFilterVariant=ContFilter  NVariant=InternalParameters  NCopyVariant=Disabled  FilterICVariant=InternalICsFilter  IntegratorICVariant=InternalICs  ExternalResetVariant=Disabled  TRSumVariant=Passthrough  SumFdbkVariant=Disabled  SumVariant=Sum_PID  TsampFilterVariant=InternalTs  TsampNgainVariant=Passthrough  TsampIntegralVariant=Passthrough  ExternalSaturationOutDataTypeStr=Inherit: Same as second input
  PID Controller4 : pid_lib/PID Controller  Controller=PID  Form=Parallel  TimeDomain=Continuous-time  UseExternalTs=off  SampleTime=-1  IntegratorMethod=Forward Euler  FilterMethod=Forward Euler  ControllerParametersSource=internal  P=0.5  I=0  D=0  UseFilter=on  N=100  TunerSelectOption=Transfer Function Based (PID Tuner App)  InitialConditionSource=internal  InitialConditionForIntegrator=0  InitialConditionForFilter=0  DifferentiatorICPrevScaledInput=0  ExternalReset=none  TrackingMode=off  Kt=1  LimitOutput=on  SatLimitsSource=internal  UpperSaturationLimit=1  LowerSaturationLimit=-1  LinearizeAsGain=on  AntiWindupMode=none  Kb=1  POutMin=[]  POutMax=[]  IOutMin=[]  IOutMax=[]  DOutMin=[]  DOutMax=[]  NOutMin=[]  NOutMax=[]  SumOutMin=[]  SumOutMax=[]  SaturationOutMin=[]  SaturationOutMax=[]  PParamMin=[]  PParamMax=[]  IParamMin=[]  IParamMax=[]  DParamMin=[]  DParamMax=[]  NParamMin=[]  NParamMax=[]  KbParamMin=[]  KbParamMax=[]  KtParamMin=[]  KtParamMax=[]  KbOutMin=[]  KbOutMax=[]  KtOutMin=[]  KtOutMax=[]  IntegratorOutMin=[]  IntegratorOutMax=[]  FilterOutMin=[]  FilterOutMax=[]  SumI1OutMin=[]  SumI1OutMax=[]  SumI2OutMin=[]  SumI2OutMax=[]  SumI3OutMin=[]  SumI3OutMax=[]  SumI4OutMin=[]  SumI4OutMax=[]  SumDOutMin=[]  SumDOutMax=[]  DifferentiatorOutMin=[]  DifferentiatorOutMax=[]  FilterDiffOutCoefMin=[]  FilterDiffOutCoefMax=[]  ReciprocalOutMin=[]  ReciprocalOutMax=[]  SumDenOutMin=[]  SumDenOutMax=[]  SumNumOutMin=[]  SumNumOutMax=[]  DivideOutMin=[]  DivideOutMax=[]  UdiffTsProdOutMin=[]  UdiffTsProdOutMax=[]  NTsProdOutMin=[]  NTsProdOutMax=[]  UintegralTsProdOutMin=[]  UintegralTsProdOutMax=[]  UngainTsProdOutMin=[]  UngainTsProdOutMax=[]  IntegratorContinuousStateAttributes=''  IntegratorStateMustResolveToSignalObject=off  IntegratorRTWStateStorageClass=Auto  FilterContinuousStateAttributes=''  FilterStateMustResolveToSignalObject=off  FilterRTWStateStorageClass=Auto  ParallelPVariant=InternalParameters  IdealPVariant=Disabled  IVariant=InternalParameters  DVariant=InternalParameters  IntegratorVariant=Continuous  SatVariant=Enabled  AWVariant=Passthrough  PCopyVariant=Disabled  TRVariant=Disabled  FdbkBlocksVariant=Forward  IdealPFdbkVariant=Disabled  SatFdbkVariant=Disabled  DerivativeFilterVariant=ContFilter  NVariant=InternalParameters  NCopyVariant=Disabled  FilterICVariant=InternalICsFilter  IntegratorICVariant=InternalICs  ExternalResetVariant=Disabled  TRSumVariant=Passthrough  SumFdbkVariant=Disabled  SumVariant=Sum_PID  TsampFilterVariant=InternalTs  TsampNgainVariant=Passthrough  TsampIntegralVariant=Passthrough  ExternalSaturationOutDataTypeStr=Inherit: Same as second input
  tao_Y : Outport
  wires:
  PID Controller1/1 -> tao_Y/1  "tao_Y"
  PID Controller4/1 -> Add5/2  "vd"
  Add5/1 -> PID Controller1/1
  dy/1 -> PID Controller4/1
  v/1 -> Add5/1  "v"

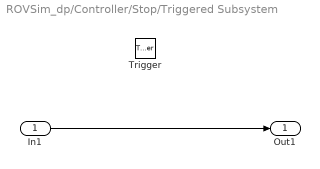
== system ROVSim_dp/Controller/Stop/Triggered Subsystem ==
  In1 : Inport
  Trigger : TriggerPort  TriggerType=falling  VariantControl=Variant
  Out1 : Outport  InitialOutput=1000
  wires:
  In1/1 -> Out1/1

== system ROVSim_dp/Controller/Stop/Triggered Subsystem1 ==
  Trigger : TriggerPort  VariantControl=Variant
  Constant : Constant
  Stop Simulation : Stop
  wires:
  Constant/1 -> Stop Simulation/1

== matlab function ROVSim_dp/Kinematics/MATLAB Function ==
  data: flowDir input; flowu output; flowVel input; psi input; flowv output
function [flowu,flowv] = fcn(flowDir,flowVel,psi)
dAngle = flowDir - psi;
if dAngle > 2*pi
    dAngle = dAngle-2*pi;
elseif dAngle<0
    dAngle = dAngle+2*pi;
end
flowu = flowVel*cos(dAngle);
flowv = flowVel*sin(dAngle);

== matlab function ROVSim_dp/Thrusters/MATLAB Function ==
  data: u input; y output; up input; low input
function y = fcn(u,up,low)
y = u;
for i=1:8
    if y(i) < up && y(i) >low
        y(i) = 0;
    end
end
end

== matlab function ROVSim_dp/Controller/MATLAB Function ==
  data: dp input; Yaw input; dx output; dy output; dz output
function [dx,dy,dz] = fcn(dp,Yaw)
psi = Yaw/180*pi;
y = [cos(psi) sin(psi); -sin(psi) cos(psi)]*dp(1:2);
dx = y(1);
dy = y(2);
dz = dp(3);
